simulink model "ADRC_control"  (R2016a)
settings: Solver=ode1  StartTime=0.0  StopTime=inf  FixedStep=0.01  RelTol=1e-3
undefined symbols (not defined in the file or in its folder): magnitude, serial
libraries: instrumentlib x3, simulink x2, dspfdesign x1
settings Model: Creator=lsr  LastModifiedBy=lsr

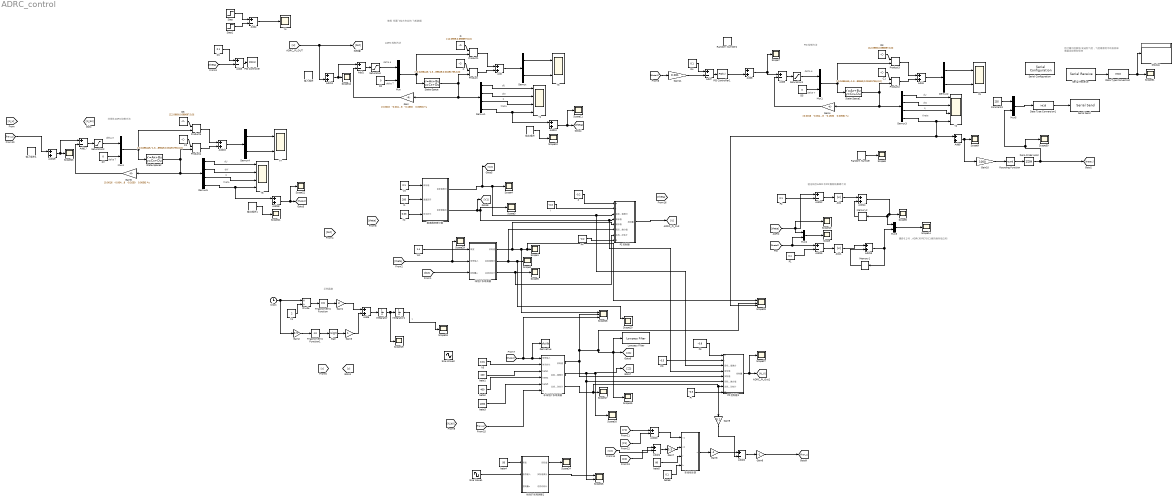
== system ADRC_control ==
  note: 将计算出的数值 发送到飞控，飞控再原封不动发回来
      | 需要添加零阶保持
  note: 验证线性ADRC和PID跟踪效果哪个好
  note: 跟踪0.1时，ADRC和PID与0.1差的绝对值之和
  note: 示例函数
  note: ADRC控制方法
  note: PID控制方法
  note: y
  note: 使用 何磊飞控大作业的 飞机数据
  note: theta
  note: q
  note: dW
  note: dU
  note: delte T
  note: delta e
  note: theta
  note: q
  note: dW
  note: dU
  note: delte T
  note: delta e
  note: 非线性ADRC控制方法
  note: theta
  note: q
  note: dW
  note: dU
  note: delte T
  note: delta e
  Abs : Abs
  Abs1 : Abs
  Add{,4,6,8..11,13..14,16,18..19} (12 alike) : Sum
  Add{1..3,5,7,12,15,17,20..22} (11 alike) : Sum  Inputs=+-
  C : Constant  Value=[-0.0498445,-1.35067,4.39526,0;-0.000189849,0.00491755,0,0]
  C1 : Constant  Value=[-0.0498445,-1.35067,4.39526,0;-0.000189849,0.00491755,0,0]
  C2 : Constant  Value=[-0.0498445,-1.35067,4.39526,0;-0.000189849,0.00491755,0,0]
  Clock : Clock
  Constant3 : Constant  Value=255
  D : Constant  Value=[12.0969,0.698697;0,0]
  D1 : Constant  Value=0.1
  D2 : Constant  Value=0
  D3 : Constant  Value=[12.0969,0.698697;0,0]
  D4 : Constant  Value=0.1
  D5 : Constant  Value=0
  D6 : Constant  Value=[12.0969,0.698697;0,0]
  D7 : Constant  Value=0
  Data Type Conversion : DataTypeConversion  OutDataTypeStr=int16
  Data Type Conversion1 : DataTypeConversion  OutDataTypeStr=int16
  Demux : Demux  Outputs=2
  Demux1 : Demux
  Demux2 : Demux  Outputs=2
  Demux3 : Demux
  Demux4 : Demux  Outputs=2
  Demux5 : Demux
  Derivative : Derivative
  Display : Display
  Divide : Product  Inputs=*/
  Gain : Gain  Gain="[0.0016   -0.0048   -0.1630    0.0056]"  Multiplication=Matrix(K*u)
  Gain1 : Gain  Gain=3
  Gain10 : Gain  Gain=1000
  Gain11 : Gain  Gain=0.001
  Gain2 : Gain  Gain=0.5
  Gain3 : Gain
  Gain4 : Gain  Gain="[0.0016   -0.0048   -0.1630    0.0056]"  Multiplication=Matrix(K*u)
  Gain5 : Gain  Gain="[0.0016   -0.0048   -0.1630    0.0056]"  Multiplication=Matrix(K*u)
  Gain6 : Gain  Gain=-1
  Gain7 : Gain  Gain=0.3
  Gain8 : Gain  Gain=-1
  Gain9 : Gain  Gain=0.1
  I : Constant  Value=-0.3
  Integrator : Integrator
  Integrator1 : Integrator
  Lowpass Filter : dspfdesign/Lowpass Filter  FilterType=FIR  DesignForMinimumOrder=on  FilterOrder=50  PassbandFrequency=2  StopbandFrequency=4  PassbandRipple=0.1  StopbandAttenuation=80  InheritSampleRate=off  SampleRate=10  roundingMode=Floor  coeffsDataTypeStr=fixdt(1,16)  SimulateUsing=Interpreted execution
  Memory1 : Memory
  Memory2 : Memory
  Mux{,1..5} (6 alike) : Mux  Inputs=2
  P : Constant  Value=-0.2
  P1 : Constant  Value=0.1
  P2 : Constant  Value=0.1
  P3 : Constant  Value=-0.8
  P4 : Constant  Value=-0.2
  PD : Constant  Value=-0.5
  PD控制器 : Subsystem
  PD控制器1 : Subsystem
  PI : Constant  Value=-0.5
  PID Controller : simulink/Continuous/PID Controller  Controller=PID  TimeDomain=Continuous-time  SampleTime=-1  IntegratorMethod=Forward Euler  FilterMethod=Forward Euler  Form=Parallel  UseFilter=on  ControllerParametersSource=internal  P=-1.2  I=-0.5  D=0  N=0  InitialConditionSource=internal  InitialConditionForIntegrator=0  InitialConditionForFilter=0  ExternalReset=none  LimitOutput=off  UpperSaturationLimit=inf  LowerSaturationLimit=-inf  LinearizeAsGain=on  AntiWindupMode=none  Kb=1  TrackingMode=off  Kt=1  PParamMin=[]  PParamMax=[]  IParamMin=[]  IParamMax=[]  DParamMin=[]  DParamMax=[]  NParamMin=[]  NParamMax=[]  KbParamMin=[]  KbParamMax=[]  KtParamMin=[]  KtParamMax=[]  POutMin=[]  POutMax=[]  IOutMin=[]  IOutMax=[]  DOutMin=[]  DOutMax=[]  NOutMin=[]  NOutMax=[]  KbOutMin=[]  KbOutMax=[]  KtOutMin=[]  KtOutMax=[]  IntegratorOutMin=[]  IntegratorOutMax=[]  FilterOutMin=[]  FilterOutMax=[]  SumOutMin=[]  SumOutMax=[]  SumI1OutMin=[]  SumI1OutMax=[]  SumI2OutMin=[]  SumI2OutMax=[]  SumI3OutMin=[]  SumI3OutMax=[]  SumDOutMin=[]  SumDOutMax=[]  SaturationOutMin=[]  SaturationOutMax=[]  IntegratorContinuousStateAttributes=''  IntegratorStateMustResolveToSignalObject=off  IntegratorRTWStateStorageClass=Auto  FilterContinuousStateAttributes=''  FilterStateMustResolveToSignalObject=off  FilterRTWStateStorageClass=Auto  DifferentiatorICPrevScaledInput=0  DifferentiatorOutMin=[]  DifferentiatorOutMax=[]
  PID Controller1 : simulink/Continuous/PID Controller  Controller=PID  TimeDomain=Continuous-time  SampleTime=-1  IntegratorMethod=Forward Euler  FilterMethod=Forward Euler  Form=Parallel  UseFilter=on  ControllerParametersSource=internal  P=-1.6  I=-0.5  D=-0.5  N=0  InitialConditionSource=internal  InitialConditionForIntegrator=0  InitialConditionForFilter=0  ExternalReset=none  LimitOutput=off  UpperSaturationLimit=inf  LowerSaturationLimit=-inf  LinearizeAsGain=on  AntiWindupMode=none  Kb=1  TrackingMode=off  Kt=1  PParamMin=[]  PParamMax=[]  IParamMin=[]  IParamMax=[]  DParamMin=[]  DParamMax=[]  NParamMin=[]  NParamMax=[]  KbParamMin=[]  KbParamMax=[]  KtParamMin=[]  KtParamMax=[]  POutMin=[]  POutMax=[]  IOutMin=[]  IOutMax=[]  DOutMin=[]  DOutMax=[]  NOutMin=[]  NOutMax=[]  KbOutMin=[]  KbOutMax=[]  KtOutMin=[]  KtOutMax=[]  IntegratorOutMin=[]  IntegratorOutMax=[]  FilterOutMin=[]  FilterOutMax=[]  SumOutMin=[]  SumOutMax=[]  SumI1OutMin=[]  SumI1OutMax=[]  SumI2OutMin=[]  SumI2OutMax=[]  SumI3OutMin=[]  SumI3OutMax=[]  SumDOutMin=[]  SumDOutMax=[]  SaturationOutMin=[]  SaturationOutMax=[]  IntegratorContinuousStateAttributes=''  IntegratorStateMustResolveToSignalObject=off  IntegratorRTWStateStorageClass=Auto  FilterContinuousStateAttributes=''  FilterStateMustResolveToSignalObject=off  FilterRTWStateStorageClass=Auto  DifferentiatorICPrevScaledInput=0  DifferentiatorOutMin=[]  DifferentiatorOutMax=[]
  Product{,1..5} (6 alike) : Product  Multiplication=Matrix(*)
  Random Number : RandomNumber  Variance=0.000001  SampleTime=0.01
  Random Number2 : RandomNumber  Variance=0.00005  SampleTime=0.01
  Rounding Function : Rounding  Operator=round
  Saturation : Saturate  UpperLimit=30/180*pi  LowerLimit=-30/180*pi
  Saturation1 : Saturate  UpperLimit=30/180*pi  LowerLimit=-30/180*pi
  Saturation2 : Saturate  UpperLimit=30/180*pi  LowerLimit=-30/180*pi
  Scope{,1..19,21..24,27,29..31} (28 alike) : Scope
  Scope20 : Scope  NumInputPorts=3
  Scope25 : Scope  NumInputPorts=2
  Scope26 : Scope  NumInputPorts=3
  Scope28 : Scope  NumInputPorts=3
  Serial Configuration : instrumentlib/Serial Configuration  Priority=-200000  ComPortMenu=COM20  ComPort=COM20  ObjConstructor=serial('COM20');  BaudRate=9600  DataBits=8  Parity=none  StopBits=1  FlowControl=none  Timeout=0.01  ByteOrder=BigEndian
  Serial Receive : instrumentlib/Serial Receive  ComPortMenu=COM20  ComPort=COM20  ObjConstructor=serial('COM20');  Terminator=<none>  DataSize=[1 1]  DataType=int16  EnableBlockingMode=on  ActionDataUnavailable=Output last received value  CustomValue=0  SampleTime=0.01
  Serial Send : instrumentlib/Serial Send  ComPortMenu=COM20  ComPort=COM20  ObjConstructor=serial('COM20');  Terminator=<none>  EnableBlockingMode=on
  Sign : Signum
  Sine Wave1 : Sin  SampleTime=0
  Sine Wave2 : Sin  SampleTime=0
  State-Space : StateSpace  A=[-0.0153803,0.0439192,-7.83906,-9.80253;-0.0438131,-1.32042,203.051,-0.378441;0.00123923,0.00621593,-0.903074,0;0,0,1,0]  B=[2.07005,9.57054;-88.0560,0;-20.5780,-0.143558;0,0]  C=[1,0,0,0;0,1,0,0;0,0,1,0;0,0,0,1]  D=[0,0;0,0;0,0;0,0]  X0=[0,0,0,0]
  State-Space1 : StateSpace  A=[-0.0153803,0.0439192,-7.83906,-9.80253;-0.0438131,-1.32042,203.051,-0.378441;0.00123923,0.00621593,-0.903074,0;0,0,1,0]  B=[2.07005,9.57054;-88.0560,0;-20.5780,-0.143558;0,0]  C=[1,0,0,0;0,1,0,0;0,0,1,0;0,0,0,1]  D=[0,0;0,0;0,0;0,0]  X0=[0,0,0,0]
  State-Space2 : StateSpace  A=[-0.0153803,0.0439192,-7.83906,-9.80253;-0.0438131,-1.32042,203.051,-0.378441;0.00123923,0.00621593,-0.903074,0;0,0,1,0]  B=[2.07005,9.57054;-88.0560,0;-20.5780,-0.143558;0,0]  C=[1,0,0,0;0,1,0,0;0,0,1,0;0,0,0,1]  D=[0,0;0,0;0,0;0,0]  X0=[0,0,0,0]
  Step : Step  After=1/180*pi  SampleTime=0
  Step1 : Step  Time=1.1  After=1/180*pi  SampleTime=0
  Trigonometric Function : Trigonometry  Operator=cos
  Trigonometric Function1 : Trigonometry
  V0 : Constant  Value=0.1
  W1 : Constant  Value=1.4
  Y1 : Scope  NumInputPorts=4
  Y2 : Scope  NumInputPorts=4
  Y3 : Scope  NumInputPorts=2
  Y4 : Scope
  Y5 : Scope  NumInputPorts=2
  Y6 : Scope  NumInputPorts=4
  Y7 : Scope  NumInputPorts=2
  Zero-Order Hold : ZeroOrderHold  SampleTime=0.01
  beta1 : Constant  Value=100
  beta2 : Constant  Value=400
  beta3 : Constant  Value=1000
  beta4 : Constant  Value=50
  beta5 : Constant  Value=80
  beta6 : Constant  Value=0.1
  h1 : Constant  Value=2
  h2 : Constant  Value=0.03
  h3 : Constant  Value=0.01
  r1 : Constant  Value=200
  最速跟踪微分器 : Subsystem
  线性扩张观测器 : Subsystem
  线性扩张观测器1 : Subsystem
  输入噪声 : RandomNumber  Variance=0.00005  SampleTime=0.01
  输入噪声1 : RandomNumber  Variance=0.00005  SampleTime=0.01
  输出噪声 : RandomNumber  Variance=0.000001  SampleTime=0.01
  输出噪声1 : RandomNumber  Variance=0.000001  SampleTime=0.01
  非线性反馈 : MATLAB Function  TreatAsAtomicUnit=on
  非线性扩张观测器 : Subsystem
  wires:
  D/1 -> Product1/1
  Product/1 -> Add/2
  Mux/1 -> Product1/2, State-Space/1
  Add/1 -> Demux/1
  Product1/1 -> Add/1
  C/1 -> Product/1
  Add1/1 -> Saturation/1
  Gain/1 -> Add1/2
  D2/1 -> Mux/2
  State-Space/1 -> Demux1/1, Gain/1, Product/2
  Demux1/1 -> Y1/1
  Demux1/2 -> Y1/2
  Demux1/3 -> Y1/3
  Step/1 -> Add2/1
  Step1/1 -> Add2/2
  Demux/1 -> Y3/1
  Demux/2 -> Y3/2
  Saturation/1 -> Mux/1
  h1/1 -> Divide/2
  Divide/1 -> Trigonometric Function/1
  Trigonometric Function/1 -> Gain1/1
  Gain1/1 -> Add6/1
  Gain2/1 -> Trigonometric Function1/1
  Trigonometric Function1/1 -> Sign/1
  Sign/1 -> Gain3/1
  Gain3/1 -> Add6/2
  Add6/1 -> Integrator/1
  Integrator/1 -> Scope19/1, Integrator1/1
  Clock/1 -> Gain2/1, Divide/1
  r1/1 -> 最速跟踪微分器/2(速度因子)
  h2/1 -> 最速跟踪微分器/3(时间步长)
  最速跟踪微分器/1(目标值微分) -> [V2], PD控制器1/3(目标值微分), PD控制器/3(目标值微分), Scope4/1
  最速跟踪微分器/2(目标值输出) -> [V1], PD控制器1/4(目标值), PD控制器/4(目标值), Scope3/1
  W1/1 -> 线性扩张观测器/1(带宽)
  线性扩张观测器/1(实际值) -> PD控制器/5(实际值), Scope26/1, Scope28/1, Scope1/1
  线性扩张观测器/2(实际值微分) -> PD控制器/6(实际微分值), Scope20/1, Scope2/1
  线性扩张观测器/3(总扰动估计) -> PD控制器/7(总扰动估计), Scope5/1
  P/1 -> PD控制器/1(P)
  I/1 -> PD控制器/2(I)
  PD控制器/1(控制量) -> [U]
  Add2/1 -> Y4/1
  [theta] -> Add3/2
  D1/1 -> Add3/1
  Add3/1 -> PID Controller/1
  V0/1 -> 最速跟踪微分器/1(目标值)
  D3/1 -> Product3/1
  Product2/1 -> Add4/2
  Mux1/1 -> Product3/2, State-Space1/1
  Add4/1 -> Demux2/1
  Product3/1 -> Add4/1
  C1/1 -> Product2/1
  Add5/1 -> Saturation1/1
  Gain4/1 -> Add5/2
  D5/1 -> Mux1/2
  State-Space1/1 -> Demux3/1, Gain4/1, Product2/2
  Demux3/1 -> Y2/1
  Demux3/2 -> Y2/2
  Demux3/3 -> Y2/3
  Demux3/4 -> Add9/1, Scope28/3, Y2/4
  Demux2/1 -> Y5/1
  Demux2/2 -> Y5/2
  Saturation1/1 -> Mux1/1
  Add7/1 -> PID Controller1/1
  Random Number/1 -> Scope8/1
  Add9/1 -> Gain10/1, Scope9/1
  Demux1/4 -> Add10/1, Y1/4
  输出噪声/1 -> Scope10/1
  Add10/1 -> Scope11/1, [theta]
  Add8/1 -> Scope7/1, Add5/1
  [U] -> Add11/2, [bUt]
  Add11/1 -> Add1/1, Scope12/1
  D4/1 -> Add7/1
  PID Controller1/1 -> Add8/2
  [theta] -> Add12/1, Mux2/1, Scope13/1
  [theta1] -> Add15/1, Mux2/2
  Mux2/1 -> Scope/1
  P2/1 -> Add12/2
  Add12/1 -> Abs/1
  Abs/1 -> Add14/1
  Memory2/1 -> Add14/2
  Abs1/1 -> Add13/1
  Add13/1 -> Memory1/1, Mux3/2
  Memory1/1 -> Add13/2
  Add15/1 -> Abs1/1
  P1/1 -> Add15/2
  Mux3/1 -> Scope14/1
  Add14/1 -> Scope6/1, Mux3/1, Memory2/1
  h3/1 -> 非线性扩张观测器/2(时间步长)
  beta1/1 -> 非线性扩张观测器/3(beta1)
  beta2/1 -> 非线性扩张观测器/4(beta2)
  beta3/1 -> 非线性扩张观测器/5(beta3)
  非线性扩张观测器/1(实际值) -> PD控制器1/5(实际值), Scope15/1, Lowpass Filter/1, [Z1], Scope28/2, Scope26/2
  非线性扩张观测器/2(实际值微分) -> PD控制器1/6(实际微分值), Scope25/2, [Z2], Scope16/1
  [theta] -> Scope29/1, 线性扩张观测器/2(信号输入)
  P3/1 -> PD控制器1/1(P)
  PD/1 -> PD控制器1/2(I)
  D6/1 -> Product5/1
  Product4/1 -> Add16/2
  Mux4/1 -> Product5/2, State-Space2/1
  Add16/1 -> Demux4/1
  Product5/1 -> Add16/1
  C2/1 -> Product4/1
  Add17/1 -> Saturation2/1
  Gain5/1 -> Add17/2
  D7/1 -> Mux4/2
  State-Space2/1 -> Demux5/1, Gain5/1, Product4/2
  Demux5/1 -> Y6/1
  Demux5/2 -> Y6/2
  Demux5/3 -> Y6/3
  Demux4/1 -> Y7/1
  Demux4/2 -> Y7/2
  Saturation2/1 -> Mux4/1
  Demux5/4 -> Add18/1, Y6/4
  输出噪声1/1 -> Scope21/1
  Add18/1 -> Scope22/1, [theta2]
  Add19/1 -> Add17/1, Scope23/1
  Integrator1/1 -> Scope18/1
  [bUt] -> 线性扩张观测器/3(控制量u)
  beta4/1 -> 线性扩张观测器1/1(带宽)
  Sine Wave1/1 -> 线性扩张观测器1/2(信号输入)
  线性扩张观测器1/1(实际值) -> Scope24/1
  线性扩张观测器1/2(实际值微分) -> Scope25/1
  [theta2] -> Scope26/3, Derivative/1, 非线性扩张观测器/1(信号输入)
  PD控制器1/1(控制量) -> Scope27/1, [N_U]
  P4/1 -> PD控制器/8(D)
  PI/1 -> PD控制器1/8(Pi)
  非线性扩张观测器/3(总扰动估计) -> Gain9/1, PD控制器1/7(总扰动估计), Scope17/1
  [fhan_U] -> 非线性扩张观测器/6(U)
  [V1] -> Add20/1
  [Z1] -> Add20/2
  Add20/1 -> 非线性反馈/1(x1)
  [Z2] -> Add21/2
  [V2] -> Add21/1
  Add21/1 -> Gain7/1
  beta5/1 -> 非线性反馈/3(r)
  beta6/1 -> 非线性反馈/4(h)
  非线性反馈/1(u) -> Gain8/1
  Add22/1 -> Gain6/1
  [fhan_U] -> Add19/1
  Gain7/1 -> 非线性反馈/2(x2)
  Gain8/1 -> Add22/1
  Gain6/1 -> [fhan_U]
  Gain9/1 -> Add22/2
  Gain10/1 -> Rounding Function/1
  Gain11/1 -> Add7/2
  Data Type Conversion1/1 -> Serial Send/1
  Constant3/1 -> Mux5/1
  Mux5/1 -> Data Type Conversion1/1
  Rounding Function/1 -> Zero-Order Hold/1
  Serial Receive/1 -> Data Type Conversion/1
  Zero-Order Hold/1 -> Mux5/2, Scope30/1, [theta1]
  Data Type Conversion/1 -> Display/1, Scope31/1
  [theta1] -> Gain11/1

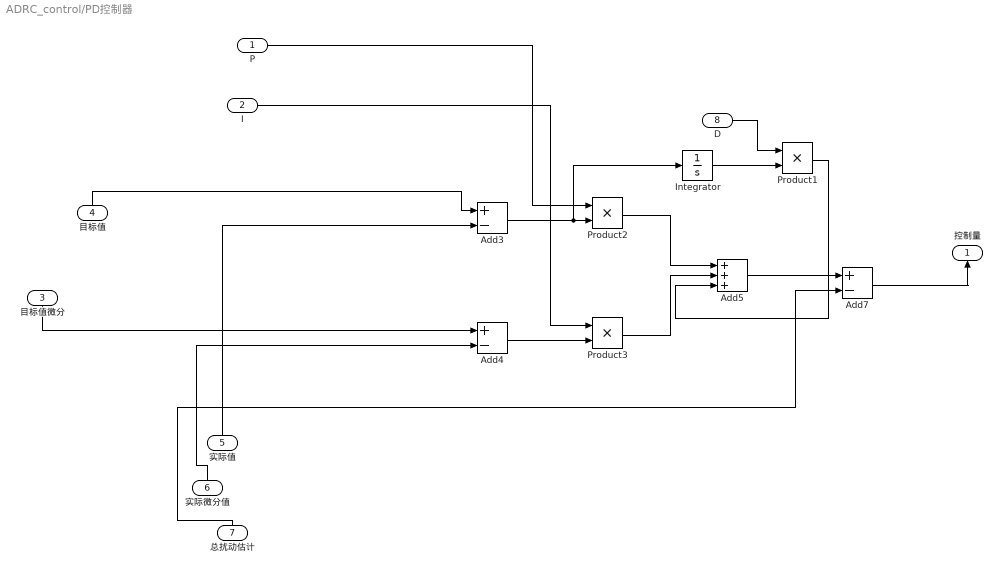
== system ADRC_control/PD控制器 ==
  P : Inport
  I : Inport  Port=2
  目标值微分 : Inport  Port=3
  目标值 : Inport  Port=4
  实际值 : Inport  Port=5
  实际微分值 : Inport  Port=6
  总扰动估计 : Inport  Port=7
  D : Inport  Port=8
  Add3 : Sum  Inputs=+-
  Add4 : Sum  Inputs=+-
  Add5 : Sum  Inputs=+++
  Add7 : Sum  Inputs=+-
  Integrator : Integrator
  Product1 : Product
  Product2 : Product
  Product3 : Product
  控制量 : Outport
  wires:
  Add7/1 -> 控制量/1
  P/1 -> Product2/1
  I/1 -> Product3/1
  Product2/1 -> Add5/1
  Add3/1 -> Integrator/1, Product2/2
  实际值/1 -> Add3/2
  实际微分值/1 -> Add4/2
  目标值微分/1 -> Add4/1
  总扰动估计/1 -> Add7/2
  目标值/1 -> Add3/1
  Product3/1 -> Add5/2
  Add5/1 -> Add7/1
  Add4/1 -> Product3/2
  Integrator/1 -> Product1/2
  D/1 -> Product1/1
  Product1/1 -> Add5/3

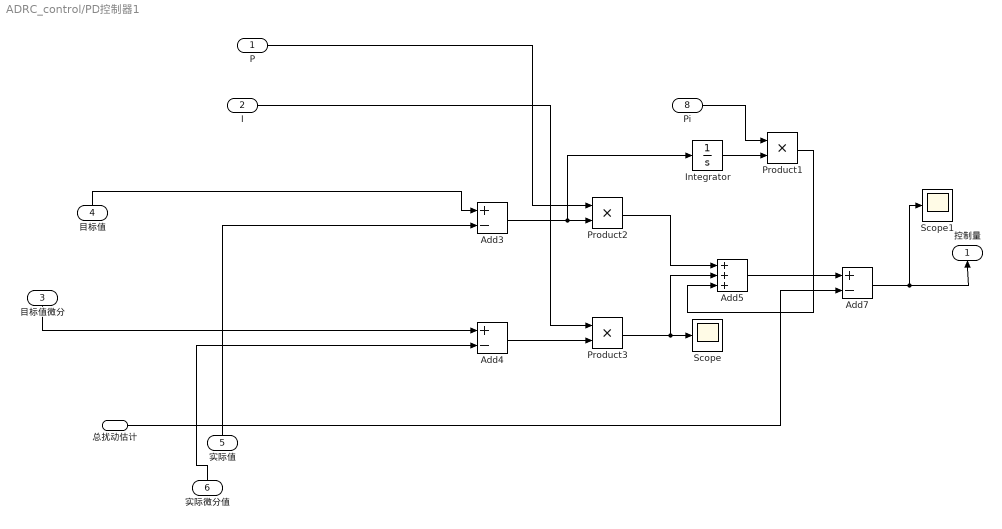
== system ADRC_control/PD控制器1 ==
  P : Inport
  I : Inport  Port=2
  目标值微分 : Inport  Port=3
  目标值 : Inport  Port=4
  实际值 : Inport  Port=5
  实际微分值 : Inport  Port=6
  总扰动估计 : Inport  Port=7
  Pi : Inport  Port=8
  Add3 : Sum  Inputs=+-
  Add4 : Sum  Inputs=+-
  Add5 : Sum  Inputs=+++
  Add7 : Sum  Inputs=+-
  Integrator : Integrator
  Product1 : Product
  Product2 : Product
  Product3 : Product
  Scope : Scope
  Scope1 : Scope
  控制量 : Outport
  wires:
  Add4/1 -> Product3/2
  Add5/1 -> Add7/1
  Product3/1 -> Scope/1, Add5/2
  目标值/1 -> Add3/1
  总扰动估计/1 -> Add7/2
  目标值微分/1 -> Add4/1
  实际微分值/1 -> Add4/2
  实际值/1 -> Add3/2
  Add3/1 -> Integrator/1, Product2/2
  Product2/1 -> Add5/1
  I/1 -> Product3/1
  P/1 -> Product2/1
  Add7/1 -> Scope1/1, 控制量/1
  Integrator/1 -> Product1/2
  Pi/1 -> Product1/1
  Product1/1 -> Add5/3

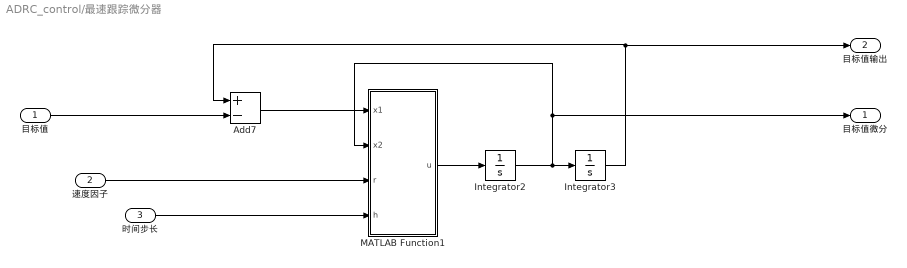
== system ADRC_control/最速跟踪微分器 ==
  目标值 : Inport
  速度因子 : Inport  Port=2
  时间步长 : Inport  Port=3
  Add7 : Sum  Inputs=+-
  Integrator2 : Integrator
  Integrator3 : Integrator
  MATLAB Function1 : MATLAB Function  TreatAsAtomicUnit=on
  目标值微分 : Outport
  目标值输出 : Outport  Port=2
  wires:
  Integrator2/1 -> 目标值微分/1, MATLAB Function1/2(x2), Integrator3/1
  Integrator3/1 -> 目标值输出/1, Add7/1
  速度因子/1 -> MATLAB Function1/3(r)
  MATLAB Function1/1(u) -> Integrator2/1
  时间步长/1 -> MATLAB Function1/4(h)
  Add7/1 -> MATLAB Function1/1(x1)
  目标值/1 -> Add7/2

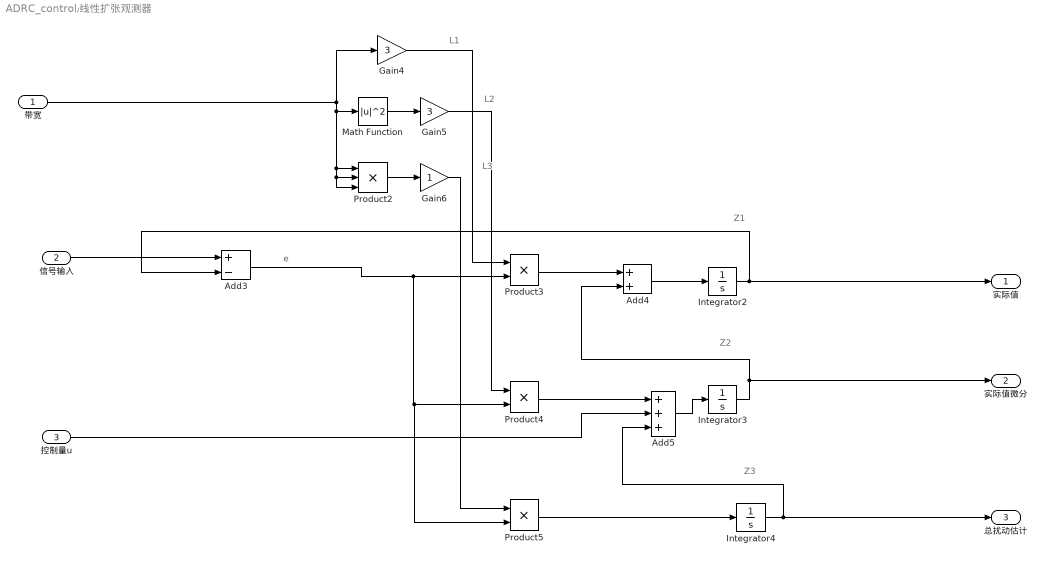
== system ADRC_control/线性扩张观测器 ==
  note: Z3
  note: Z2
  note: e
  note: L3
  note: L2
  note: L1
  note: Z1
  带宽 : Inport
  信号输入 : Inport  Port=2
  控制量u : Inport  Port=3
  Add3 : Sum  Inputs=+-
  Add4 : Sum
  Add5 : Sum  Inputs=+++
  Gain4 : Gain  Gain=3
  Gain5 : Gain  Gain=3
  Gain6 : Gain
  Integrator2 : Integrator
  Integrator3 : Integrator
  Integrator4 : Integrator
  Math Function : Math  Operator=magnitude^2  SaturateOnIntegerOverflow=on
  Product2 : Product  Inputs=3
  Product3 : Product
  Product4 : Product
  Product5 : Product
  实际值 : Outport
  实际值微分 : Outport  Port=2
  总扰动估计 : Outport  Port=3
  wires:
  信号输入/1 -> Add3/1
  Product2/1 -> Gain6/1
  Add4/1 -> Integrator2/1
  Product4/1 -> Add5/1
  Gain5/1 -> Product4/1
  Product5/1 -> Integrator4/1
  Add3/1 -> Product5/2, Product4/2, Product3/2
  Product3/1 -> Add4/1
  Integrator3/1 -> 实际值微分/1, Add4/2
  Integrator4/1 -> 总扰动估计/1, Add5/3
  Add5/1 -> Integrator3/1
  控制量u/1 -> Add5/2
  Gain6/1 -> Product5/1
  Math Function/1 -> Gain5/1
  Integrator2/1 -> 实际值/1, Add3/2
  Gain4/1 -> Product3/1
  带宽/1 -> Gain4/1, Product2/3, Product2/2, Product2/1, Math Function/1

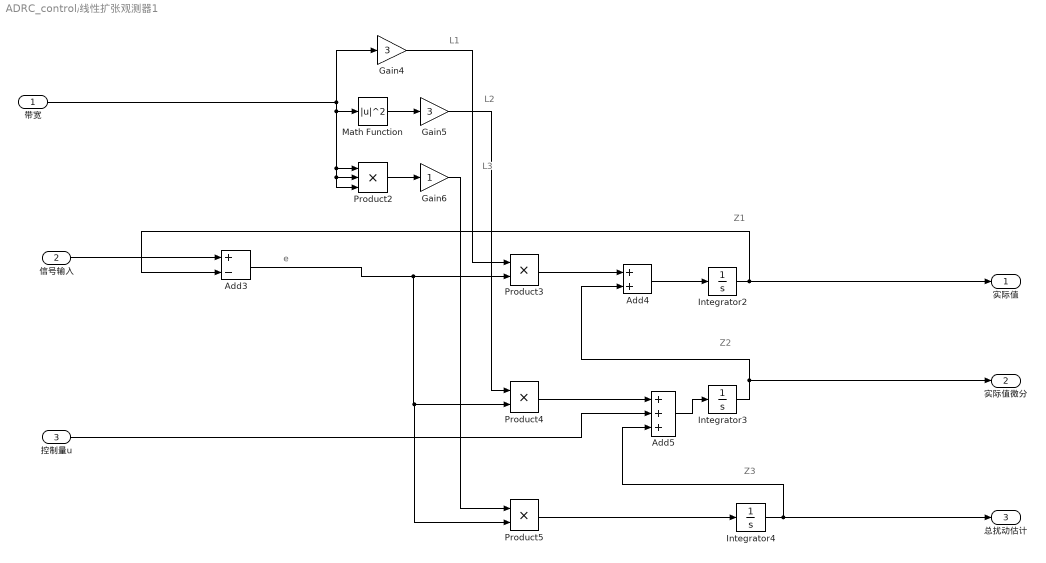
== system ADRC_control/线性扩张观测器1 ==
  note: Z1
  note: L1
  note: L2
  note: L3
  note: e
  note: Z2
  note: Z3
  带宽 : Inport
  信号输入 : Inport  Port=2
  控制量u : Inport  Port=3
  Add3 : Sum  Inputs=+-
  Add4 : Sum
  Add5 : Sum  Inputs=+++
  Gain4 : Gain  Gain=3
  Gain5 : Gain  Gain=3
  Gain6 : Gain
  Integrator2 : Integrator
  Integrator3 : Integrator
  Integrator4 : Integrator
  Math Function : Math  Operator=magnitude^2  SaturateOnIntegerOverflow=on
  Product2 : Product  Inputs=3
  Product3 : Product
  Product4 : Product
  Product5 : Product
  实际值 : Outport
  实际值微分 : Outport  Port=2
  总扰动估计 : Outport  Port=3
  wires:
  带宽/1 -> Math Function/1, Product2/1, Product2/2, Product2/3, Gain4/1
  Gain4/1 -> Product3/1
  Integrator2/1 -> Add3/2, 实际值/1
  Math Function/1 -> Gain5/1
  Gain6/1 -> Product5/1
  控制量u/1 -> Add5/2
  Add5/1 -> Integrator3/1
  Integrator4/1 -> Add5/3, 总扰动估计/1
  Integrator3/1 -> Add4/2, 实际值微分/1
  Product3/1 -> Add4/1
  Add3/1 -> Product3/2, Product4/2, Product5/2
  Product5/1 -> Integrator4/1
  Gain5/1 -> Product4/1
  Product4/1 -> Add5/1
  Add4/1 -> Integrator2/1
  Product2/1 -> Gain6/1
  信号输入/1 -> Add3/1

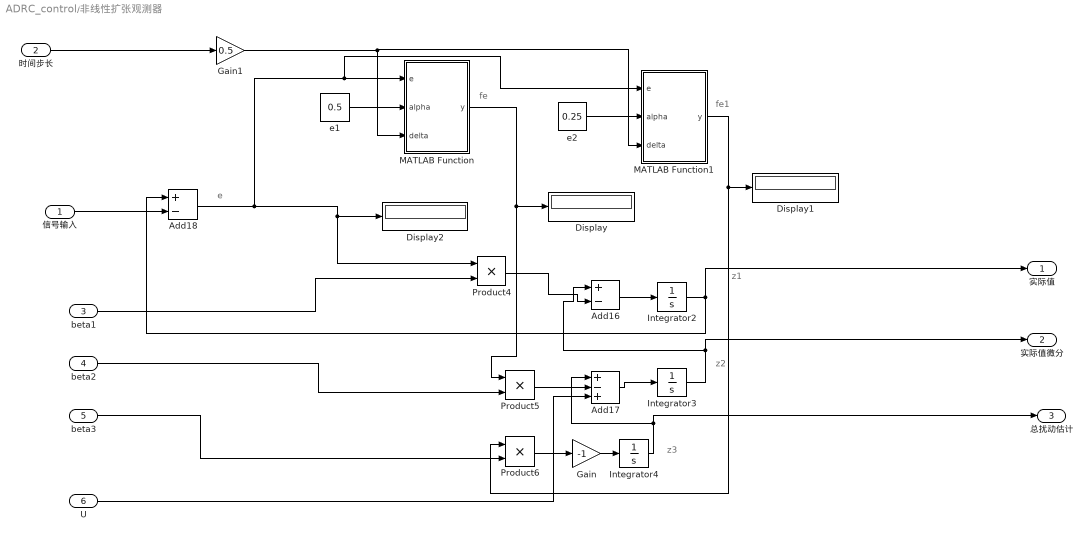
== system ADRC_control/非线性扩张观测器 ==
  note: e
  note: z3
  note: z2
  note: z1
  note: fe1
  note: fe
  信号输入 : Inport
  时间步长 : Inport  Port=2
  beta1 : Inport  Port=3
  beta2 : Inport  Port=4
  beta3 : Inport  Port=5
  U : Inport  Port=6
  Add16 : Sum  Inputs=+-
  Add17 : Sum  Inputs=+-+
  Add18 : Sum  Inputs=+-
  Display : Display
  Display1 : Display
  Display2 : Display
  Gain : Gain  Gain=-1
  Gain1 : Gain  Gain=0.5
  Integrator2 : Integrator
  Integrator3 : Integrator
  Integrator4 : Integrator
  MATLAB Function : MATLAB Function  TreatAsAtomicUnit=on
  MATLAB Function1 : MATLAB Function  TreatAsAtomicUnit=on
  Product4 : Product
  Product5 : Product
  Product6 : Product
  e1 : Constant  Value=0.5
  e2 : Constant  Value=0.25
  实际值 : Outport
  实际值微分 : Outport  Port=2
  总扰动估计 : Outport  Port=3
  wires:
  beta3/1 -> Product6/2
  beta2/1 -> Product5/2
  beta1/1 -> Product4/2
  MATLAB Function/1(y) -> Display/1, Product5/1
  e2/1 -> MATLAB Function1/2(alpha)
  Product4/1 -> Add16/2
  Product5/1 -> Add17/2
  Integrator3/1 -> 实际值微分/1, Add16/1
  时间步长/1 -> Gain1/1
  e1/1 -> MATLAB Function/2(alpha)
  Add17/1 -> Integrator3/1
  Product6/1 -> Gain/1
  Integrator4/1 -> 总扰动估计/1, Add17/1
  Add16/1 -> Integrator2/1
  MATLAB Function1/1(y) -> Display1/1, Product6/1
  Integrator2/1 -> Add18/1, 实际值/1
  Add18/1 -> MATLAB Function1/1(e), MATLAB Function/1(e), Display2/1, Product4/1
  信号输入/1 -> Add18/2
  U/1 -> Add17/3
  Gain/1 -> Integrator4/1
  Gain1/1 -> MATLAB Function1/3(delta), MATLAB Function/3(delta)

== matlab function ADRC_control/最速跟踪微分器/MATLAB Function1 ==
  data: x1 input; u output; x2 input; r input; h input
function u = fhan(x1,x2,r,h)
% x1:V1-V0  V1为实际输出值，V0为需要跟踪的值
% x2:V0的微分
% r: 速度因子
% h: 时间步长

%输出 u： 一次积分得到V0的微分，再积分得到V0。

%FHAN 最速控制综合函数
%   此处显示详细说明
%a = 0;
%u = 0;
d = r*h;
d0 = h*d;
y = x1+h*x2;
a0 = sqrt(d*d+8*r*abs(y));

if abs(y)>d0
    a = x2+(a0-d)/2*sign(y);
else
    a = x2+y/h;
end


if abs(a)>d
    u = -r*sign(a);
else
    u = -r*a/d;
end

end

== matlab function ADRC_control/非线性扩张观测器/MATLAB Function ==
  data: e input; y output; alpha input; delta input
function y = fal(e,alpha,delta)
%非线性扩张状态观测器常用的函数fal
%P202
%e:系统实际输出y和估计值z1的差
%alpha:0.5或0.25
%delta：线性段的区间长度
%#codegen
  if abs(e)>delta
      u = abs(e)^alpha * sign(e);
  else
     % u = abs(delta)^alpha * sign(delta)/delta * e;
      u = e/(delta^(1-alpha));
  end

y = u;

== matlab function ADRC_control/非线性扩张观测器/MATLAB Function1 ==
  data: e input; y output; alpha input; delta input
function y = fal(e,alpha,delta)
%非线性扩张状态观测器常用的函数fal
%P202
%e:系统实际输出y和估计值z1的差
%alpha:0.5或0.25
%delta：线性段的区间长度
%#codegen
 if abs(e)>delta
      u = abs(e)^alpha * sign(e);
  else
     % u = abs(delta)^alpha * sign(delta)/delta * e;
      u = e/(delta^(1-alpha));
  end
y = u;

== matlab function ADRC_control/非线性反馈 ==
  data: x1 input; u output; x2 input; r input; h input
function u = fhan(x1,x2,r,h)
% x1:V1-V0  V1为实际输出值，V0为需要跟踪的值
% x2:V0的微分
% r: 速度因子
% h: 时间步长

%输出 u： 一次积分得到V0的微分，再积分得到V0。

%FHAN 最速控制综合函数
%   此处显示详细说明
%a = 0;
%u = 0;
d = r*h;
d0 = h*d;
y = x1+h*x2;
a0 = sqrt(d*d+8*r*abs(y));

if abs(y)>d0
    a = x2+(a0-d)/2*sign(y);
else
    a = x2+y/h;
end


if abs(a)>d
    u = -r*sign(a);
else
    u = -r*a/d;
end

end
